simulink model "model_test"  (R2022b)
settings: Solver=VariableStepAuto  StartTime=0.0  StopTime=10.0  RelTol=1e-3
values from neighbouring files (symbols this model uses):
  Mass = 10    [matlab.m]
settings Model: Creator=Artis  LastModifiedBy=Artis

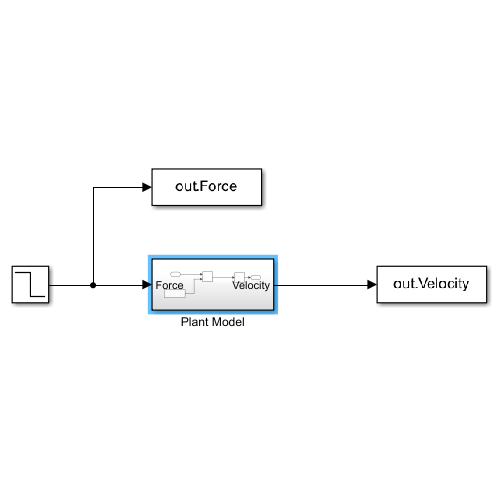
[thumbnail: Simulink's stored preview of the top-level diagram]
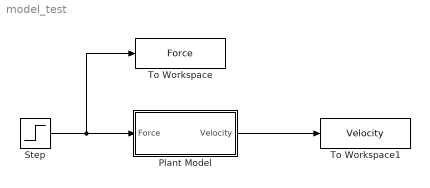
== system model_test ==
  Plant Model : Subsystem
  Step : Step  Before=1  After=0  SampleTime=0
  To Workspace : ToWorkspace  VariableName=Force  SaveFormat=Timeseries  SampleTime=-1
  To Workspace1 : ToWorkspace  VariableName=Velocity  SaveFormat=Timeseries  SampleTime=-1
  wires:
  Step/1 -> To Workspace/1, Plant Model/1(Force)
  Plant Model/1(Velocity) -> To Workspace1/1

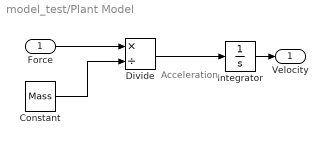
== system model_test/Plant Model ==
  note: Acceleration
  Force : Inport
  Constant : Constant  Value=Mass
  Divide : Product  Inputs=*/
  Integrator : Integrator
  Velocity : Outport
  wires:
  Force/1 -> Divide/1
  Integrator/1 -> Velocity/1
  Divide/1 -> Integrator/1
  Constant/1 -> Divide/2
